simulink model "DynmaicModel"  (R2018a)
settings: Solver=VariableStepAuto  StartTime=0.0  StopTime=1  RelTol=1e-3
undefined symbols (not defined in the file): A, B, C, D
libraries: simulink x1
settings Model: Creator=BC  LastModifiedBy=BC

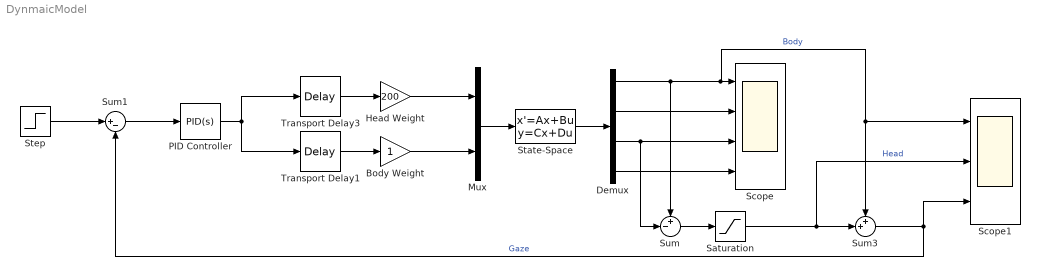
== system DynmaicModel ==
  Body Weight : Gain
  Demux : Demux
  Head Weight : Gain  Gain=200
  Mux : Mux  Inputs=2
  PID Controller : simulink/Continuous/PID Controller  Controller=PID  TimeDomain=Continuous-time  SampleTime=-1  IntegratorMethod=Forward Euler  FilterMethod=Forward Euler  Form=Parallel  UseFilter=on  ControllerParametersSource=internal  P=3.97128367896402e-07  I=4.04823407453199e-06  D=9.57444732457901e-09  N=2462.617874973  InitialConditionSource=internal  InitialConditionForIntegrator=0  InitialConditionForFilter=0  ExternalReset=none  LimitOutput=off  UpperSaturationLimit=inf  LowerSaturationLimit=-inf  LinearizeAsGain=on  AntiWindupMode=none  Kb=1  TrackingMode=off  Kt=1  PParamMin=[]  PParamMax=[]  IParamMin=[]  IParamMax=[]  DParamMin=[]  DParamMax=[]  NParamMin=[]  NParamMax=[]  KbParamMin=[]  KbParamMax=[]  KtParamMin=[]  KtParamMax=[]  POutMin=[]  POutMax=[]  IOutMin=[]  IOutMax=[]  DOutMin=[]  DOutMax=[]  NOutMin=[]  NOutMax=[]  KbOutMin=[]  KbOutMax=[]  KtOutMin=[]  KtOutMax=[]  IntegratorOutMin=[]  IntegratorOutMax=[]  FilterOutMin=[]  FilterOutMax=[]  SumOutMin=[]  SumOutMax=[]  SumI1OutMin=[]  SumI1OutMax=[]  SumI2OutMin=[]  SumI2OutMax=[]  SumI3OutMin=[]  SumI3OutMax=[]  SumDOutMin=[]  SumDOutMax=[]  SaturationOutMin=[]  SaturationOutMax=[]  IntegratorContinuousStateAttributes=''  IntegratorStateMustResolveToSignalObject=off  IntegratorRTWStateStorageClass=Auto  FilterContinuousStateAttributes=''  FilterStateMustResolveToSignalObject=off  FilterRTWStateStorageClass=Auto  DifferentiatorICPrevScaledInput=0  DifferentiatorOutMin=[]  DifferentiatorOutMax=[]  FilterDiffOutCoefMin=[]  FilterDiffOutCoefMax=[]  SumDenOutMin=[]  SumDenOutMax=[]  SumNumOutMin=[]  SumNumOutMax=[]  ReciprocalOutMin=[]  ReciprocalOutMax=[]  DivideOutMin=[]  DivideOutMax=[]  TunerSelectOption=Transfer Function Based (PID Tuner App)
  Saturation : Saturate  UpperLimit=17  LowerLimit=-17
  Scope : Scope  NumInputPorts=4
  Scope1 : Scope  NumInputPorts=3
  State-Space : StateSpace  A=A  B=B  C=C  D=D  InitialCondition=0
  Step : Step  Time=0.1  SampleTime=0
  Sum : Sum  Inputs=+-|
  Sum1 : Sum  Inputs=|+-
  Sum3 : Sum  Inputs=++|
  Transport Delay1 : TransportDelay  DelayTime=0
  Transport Delay3 : TransportDelay  DelayTime=0
  wires:
  Mux/1 -> State-Space/1
  State-Space/1 -> Demux/1
  Transport Delay1/1 -> Body Weight/1
  Transport Delay3/1 -> Head Weight/1
  Head Weight/1 -> Mux/1
  Body Weight/1 -> Mux/2
  PID Controller/1 -> Transport Delay3/1, Transport Delay1/1
  Sum1/1 -> PID Controller/1
  Step/1 -> Sum1/1
  Demux/1 -> Sum3/1, Scope1/1, Scope/1, Sum/1  "Body"
  Demux/3 -> Scope/3, Sum/2
  Demux/2 -> Scope/2
  Demux/4 -> Scope/4
  Sum/1 -> Saturation/1
  Saturation/1 -> Scope1/2, Sum3/2  "Head"
  Sum3/1 -> Sum1/2, Scope1/3  "Gaze"
